simulink model "ex1"  (R2018b)
settings: Solver=VariableStepAuto  StartTime=0.0  StopTime=10  RelTol=1e-3
settings Model: Creator=frodan  LastModifiedBy=frodan

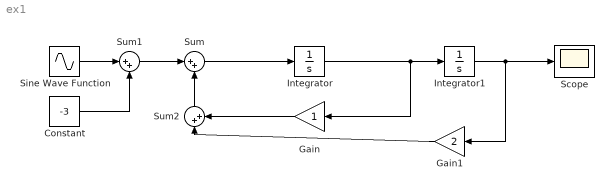
== system ex1 ==
  Constant : Constant  Value=-3
  Gain : Gain
  Gain1 : Gain  Gain=2
  Integrator : Integrator  InitialCondition=2
  Integrator1 : Integrator  InitialCondition=5
  Scope : Scope
  Sine Wave Function : Sin  Frequency=2  SampleTime=0
  Sum : Sum  Inputs=|++
  Sum1 : Sum  Inputs=|++
  Sum2 : Sum  Inputs=|++
  wires:
  Sum/1 -> Integrator/1
  Integrator/1 -> Gain/1, Integrator1/1
  Integrator1/1 -> Gain1/1, Scope/1
  Constant/1 -> Sum1/2
  Sine Wave Function/1 -> Sum1/1
  Sum1/1 -> Sum/1
  Sum2/1 -> Sum/2
  Gain/1 -> Sum2/2
  Gain1/1 -> Sum2/1
